simulink model "random_communication_loss"  (R2018a)
settings: Solver=VariableStepAuto  StartTime=0.0  StopTime=10.0  RelTol=1e-3
settings Model: Creator=blond  LastModifiedBy=daniel

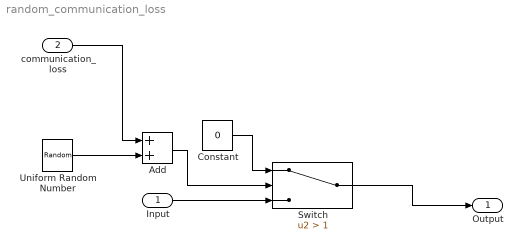
== system random_communication_loss ==
  Input : Inport
  communication_loss : Inport  Port=2
  Add : Sum
  Constant : Constant  Value=0
  Switch : Switch  Criteria=u2 > Threshold  Threshold=1
  Uniform Random Number : UniformRandomNumber  Minimum=0  Maximum=999  Seed=1337  SampleTime=0.1
  Output : Outport
  wires:
  Uniform Random Number/1 -> Add/2
  Constant/1 -> Switch/1
  Input/1 -> Switch/3
  Switch/1 -> Output/1
  communication_loss/1 -> Add/1
  Add/1 -> Switch/2
